simulink model "SDRPart2"  (R2023a)
settings: Solver=FixedStepAuto  StartTime=0.0  StopTime=0.01  FixedStep=1.25e-8  RelTol=1e-3
values from neighbouring files (symbols this model uses):
  cos_out_padded = paddedVectorForCIC(cos_out, 4096)    [SDR.m]
  sin_out_padded = paddedVectorForCIC(sin_out, 4096)    [SDR.m]
undefined symbols (not defined in the file or in its folder): fdesignblkfcn, gcbh
libraries: dspmlti4 x2
settings Model: Creator=User  LastModifiedBy=User

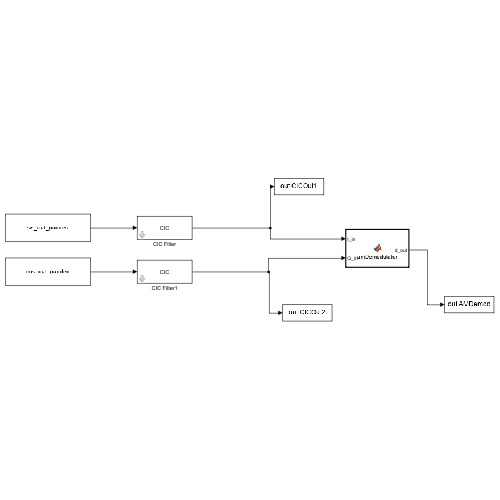
[thumbnail: Simulink's stored preview of the top-level diagram]
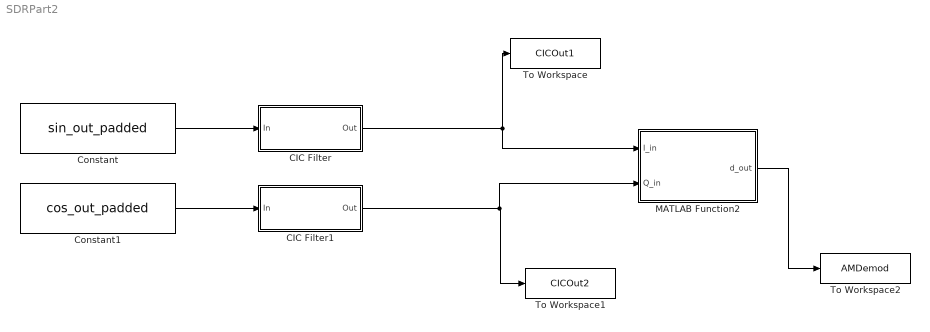
== system SDRPart2 ==
  CIC Filter : Subsystem  DialogController=fdesignblkfcn  InitFcn=fdesignblkfcn(gcbh, {'InitFcn'});  mask(CIC Filter){}
      mask help: dsp:DSPFilterDesignBlockDialog:CICFdesign_MaskDesc
      settings: CopyFcn=fdesignblkfcn(gcbh, {'CopyFcn'});
      mask Help: helpview(mapfilelocation('dsp'), 'dspcicfilter');
      mask Display: disp('CIC')
  CIC Filter1 : Subsystem  DialogController=fdesignblkfcn  InitFcn=fdesignblkfcn(gcbh, {'InitFcn'});  mask(CIC Filter){}
      mask help: dsp:DSPFilterDesignBlockDialog:CICFdesign_MaskDesc
      settings: CopyFcn=fdesignblkfcn(gcbh, {'CopyFcn'});
      mask Help: helpview(mapfilelocation('dsp'), 'dspcicfilter');
      mask Display: disp('CIC')
  Constant : Constant  Value=sin_out_padded
  Constant1 : Constant  Value=cos_out_padded
  MATLAB Function2 : MATLAB Function  TreatAsAtomicUnit=on
  To Workspace : ToWorkspace  VariableName=CICOut1  SaveFormat=Structure With Time  SampleTime=-1
  To Workspace1 : ToWorkspace  VariableName=CICOut2  SaveFormat=Structure With Time  SampleTime=-1
  To Workspace2 : ToWorkspace  VariableName=AMDemod  SaveFormat=Structure With Time  SampleTime=-1
  wires:
  CIC Filter/1(Out) -> MATLAB Function2/1(I_in), To Workspace/1
  CIC Filter1/1(Out) -> MATLAB Function2/2(Q_in), To Workspace1/1
  Constant/1 -> CIC Filter/1(In)
  Constant1/1 -> CIC Filter1/1(In)
  MATLAB Function2/1(d_out) -> To Workspace2/1

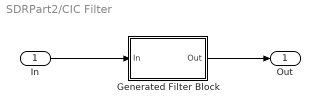
== system SDRPart2/CIC Filter ==
  In : Inport
  Generated Filter Block : Subsystem  Tag=BlockMethodSubSystem
  Out : Outport  VectorParamsAs1DForOutWhenUnconnected=off
  wires:
  In/1 -> Generated Filter Block/1(In)
  Generated Filter Block/1(Out) -> Out/1

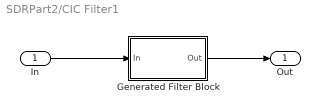
== system SDRPart2/CIC Filter1 ==
  In : Inport
  Generated Filter Block : Subsystem  Tag=BlockMethodSubSystem
  Out : Outport  VectorParamsAs1DForOutWhenUnconnected=off
  wires:
  In/1 -> Generated Filter Block/1(In)
  Generated Filter Block/1(Out) -> Out/1

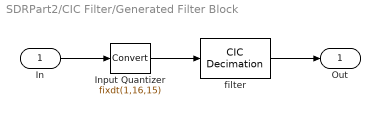
== system SDRPart2/CIC Filter/Generated Filter Block ==
  In : Inport
  Input Quantizer : DataTypeConversion  OutDataTypeStr=fixdt(1,16,15)  RndMeth=Round
  filter : dspmlti4/CIC Decimation  filtFrom=Dialog parameters  filtobj=CICDECIM  ftype=Decimator  R=4096  M=1  N=2  filterInternals=Full precision  BPS=[40 40 40 40]  FLPS=[15 15 15 15]  outputWordLength=40  outputFracLength=15  launchFVT=off  framing=Maintain input frame rate  RateOptions=Enforce single-rate processing
  Out : Outport
  wires:
  In/1 -> Input Quantizer/1
  Input Quantizer/1 -> filter/1
  filter/1 -> Out/1

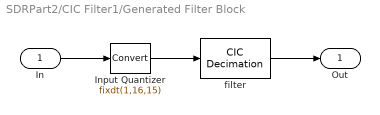
== system SDRPart2/CIC Filter1/Generated Filter Block ==
  In : Inport
  Input Quantizer : DataTypeConversion  OutDataTypeStr=fixdt(1,16,15)  RndMeth=Round
  filter : dspmlti4/CIC Decimation  filtFrom=Dialog parameters  filtobj=CICDECIM  ftype=Decimator  R=4096  M=1  N=2  filterInternals=Full precision  BPS=[40 40 40 40]  FLPS=[15 15 15 15]  outputWordLength=40  outputFracLength=15  launchFVT=off  framing=Maintain input frame rate  RateOptions=Enforce single-rate processing
  Out : Outport
  wires:
  In/1 -> Input Quantizer/1
  Input Quantizer/1 -> filter/1
  filter/1 -> Out/1

== matlab function SDRPart2/MATLAB Function2 ==
  data: I_in input; d_out output; Q_in input
function d_out = amDemodulator(I_in, Q_in)
    % amDemodulator Calculates the amplitude of a signal given its I and Q components.
    % Utilizes the sqrt function directly for simplicity and precision.

    % Calculate the squares of I and Q components
    ISquare = double(I_in).^2;
    QSquare = double(Q_in).^2;

    % Calculate the square root of the sum of the squares
    magnitude = sqrt(ISquare + QSquare);

    temp = squeeze(magnitude);

    d_out = mean(temp, 3);

    d_out = squeeze(d_out);

end
